simulink model "RLC"  (R2017b)
settings: Solver=VariableStepAuto  StartTime=0.0  StopTime=10  FixedStep=0.01  RelTol=1e-6
values from neighbouring files (symbols this model uses):
  C = 200*1e-1    (= 20)    [RLC_setting.m]
  L = 1/(C*w^2)+R/w*tan(w*tau)    [RLC_setting.m]
  R = v0*cos(w*tau)/I0    [RLC_setting.m]
  T = 1    [RLC_setting.m]
  v0 = 1    [RLC_setting.m]
  w = 2*pi/T    (= 6.28318530718)    [RLC_setting.m]
settings Model: Creator=atamo_000  LastModifiedBy=atamo_000

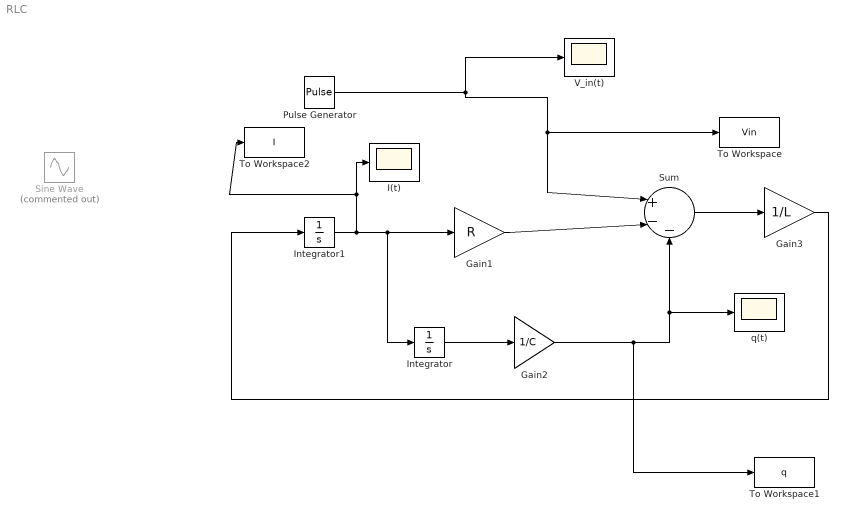
== system RLC ==
  Gain1 : Gain  Gain=R
  Gain2 : Gain  Gain=1/C
  Gain3 : Gain  Gain=1/L
  I(t) : Scope
  Integrator : Integrator
  Integrator1 : Integrator
  Pulse Generator : DiscretePulseGenerator  PulseType=Time based  Period=T  PulseWidth=20
  Sine Wave : Sin  Commented=on  Amplitude=v0  Frequency=w  SampleTime=0
  Sum : Sum  Inputs=|+--
  To Workspace : ToWorkspace  VariableName=Vin  SampleTime=-1
  To Workspace1 : ToWorkspace  VariableName=q  SampleTime=-1
  To Workspace2 : ToWorkspace  VariableName=I  SampleTime=-1
  V_in(t) : Scope
  q(t) : Scope
  wires:
  Gain1/1 -> Sum/2
  Integrator/1 -> Gain2/1
  Pulse Generator/1 -> Sum/1, To Workspace/1, V_in(t)/1
  Sum/1 -> Gain3/1
  Gain3/1 -> Integrator1/1
  Gain2/1 -> To Workspace1/1, Sum/3, q(t)/1
  Integrator1/1 -> To Workspace2/1, I(t)/1, Integrator/1, Gain1/1
